simulink model "PWM"  (Simulink 6.1)
settings: Solver=ode23tb  StartTime=0.0  StopTime=0.1  RelTol=1e-3
libraries: powerlib x16, powerlib_extras x4
settings Model: LastModifiedBy=Sonic
settings DebuggingCC: SolverPrmCheckMsg=warning

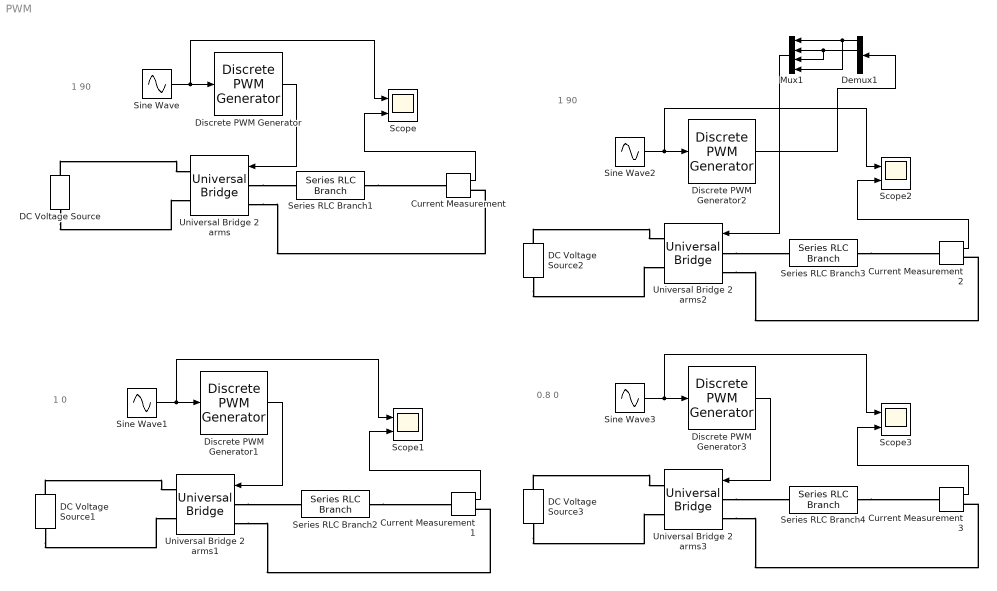
== system PWM ==
  note: 1
      | 90
  note: 1
      | 0
  note: 0.8
      | 0
  note: 1
      | 90
  Current Measurement{,1..3} (4 alike) : powerlib/Measurements/Current Measurement  PhasorSimulation=off  OutputType=Complex  PSBequivalent=0
  DC Voltage Source{,1..3} (4 alike) : powerlib/Electrical Sources/DC Voltage Source  Orientation=up  Amplitude=100  Measurements=None
  Demux1 : Demux  Orientation=left
  Discrete PWM Generator{,1..3} (4 alike) : powerlib_extras/Discrete  Control Blocks/Discrete PWM Generator  GeneratorMode="2-arm  bridge (4 pulses)"  Fc=20000  Ts=5e-6  Internal=off  mIndex=0.9  Freq=50  Phase=0
  Mux1 : Mux  Orientation=left
  Scope{,1..3} (4 alike) : Scope  NumInputPorts=2
      Scope settings: YMin=-5~-5  YMax=5~5  MaxDataPoints=500000
      Scope1 settings: YMin=-5~-5  YMax=5~5  MaxDataPoints=500000
      Scope2 settings: YMin=-5~-5  YMax=5~5  SaveName=ScopeData2  MaxDataPoints=500000
      Scope3 settings: YMin=-5~-5  YMax=5~5  SaveName=ScopeData3  MaxDataPoints=500000
  Series RLC Branch{1..4} (4 alike) : powerlib/Elements/Series RLC Branch  PhysicalDomain=powersysdomain  SubClassName=unknown  LeftPortType=p1  RightPortType=p1  LConnTagsString=__new0  RConnTagsString=__new0  Resistance=10  Inductance=0.1  Capacitance=inf  Measurements=Branch current
  Sine Wave : Sin  Frequency=100*pi  Phase=pi/2  SampleTime=0
  Sine Wave1 : Sin  Frequency=100*pi  SampleTime=0
  Sine Wave2 : Sin  Frequency=100*pi  Phase=pi/2  SampleTime=0
  Sine Wave3 : Sin  Amplitude=0.8  Frequency=100*pi  SampleTime=0
  Universal Bridge 2 arms{,1..3} (4 alike) : powerlib/Power Electronics/Universal Bridge  Orientation=left  Arms=2  SnubberResistance=10000  SnubberCapacitance=inf  Device=IGBT / Diodes  Ron=1e-4  Lon=0  ForwardVoltages="[  1  1  ]"  ForwardVoltage=.8  GTOparameters=[ 10e-6 , 20e-6 ]  IGBTparameters=[ 1e-6 , 2e-6 ]  Measurements=None
  wires:
  Sine Wave/1 -> Discrete PWM Generator/1, Scope/1
  Discrete PWM Generator/1 -> Universal Bridge 2 arms/1
  Current Measurement/1 -> Scope/2
  Sine Wave1/1 -> Scope1/1, Discrete PWM Generator1/1
  Discrete PWM Generator1/1 -> Universal Bridge 2 arms1/1
  Current Measurement1/1 -> Scope1/2
  Sine Wave2/1 -> Discrete PWM Generator2/1, Scope2/1
  Current Measurement2/1 -> Scope2/2
  Mux1/1 -> Universal Bridge 2 arms2/1
  Demux1/1 -> Mux1/4, Mux1/1
  Demux1/2 -> Mux1/3, Mux1/2
  Discrete PWM Generator2/1 -> Demux1/1
  Sine Wave3/1 -> Discrete PWM Generator3/1, Scope3/1
  Discrete PWM Generator3/1 -> Universal Bridge 2 arms3/1
  Current Measurement3/1 -> Scope3/2
  connections:
  DC Voltage Source/RConn1 -- Universal Bridge 2 arms/RConn1
  DC Voltage Source/LConn1 -- Universal Bridge 2 arms/RConn2
  Universal Bridge 2 arms/LConn1 -- Series RLC Branch1/LConn1
  Series RLC Branch1/RConn1 -- Current Measurement/LConn1
  Universal Bridge 2 arms/LConn2 -- Current Measurement/RConn1
  DC Voltage Source1/RConn1 -- Universal Bridge 2 arms1/RConn1
  DC Voltage Source1/LConn1 -- Universal Bridge 2 arms1/RConn2
  Universal Bridge 2 arms1/LConn1 -- Series RLC Branch2/LConn1
  Series RLC Branch2/RConn1 -- Current Measurement1/LConn1
  Universal Bridge 2 arms1/LConn2 -- Current Measurement1/RConn1
  DC Voltage Source2/RConn1 -- Universal Bridge 2 arms2/RConn1
  DC Voltage Source2/LConn1 -- Universal Bridge 2 arms2/RConn2
  Universal Bridge 2 arms2/LConn1 -- Series RLC Branch3/LConn1
  Series RLC Branch3/RConn1 -- Current Measurement2/LConn1
  Universal Bridge 2 arms2/LConn2 -- Current Measurement2/RConn1
  DC Voltage Source3/RConn1 -- Universal Bridge 2 arms3/RConn1
  DC Voltage Source3/LConn1 -- Universal Bridge 2 arms3/RConn2
  Universal Bridge 2 arms3/LConn1 -- Series RLC Branch4/LConn1
  Series RLC Branch4/RConn1 -- Current Measurement3/LConn1
  Universal Bridge 2 arms3/LConn2 -- Current Measurement3/RConn1
